simulink model "TSR_Scenario_002_cs"  (R2014b)
settings: Solver=ode5  SolverMode=SingleTasking  StartTime=0.0  StopTime=inf  FixedStep=1/100  RelTol=1e-3
PreLoadFcn:
  | mbxruntime.callbacks.PreLoadFcn(bdroot);
  | check_NUTS_defined;
  | 
  | assignin('base',['model_closed_' bdroot],false);
  | 
  | addpath('../includes_TSR/includes_TSR');
  | 
  | switch version('-release')
  | case {'2010a', '2010b', '2011a'}
  | addpath('../includes_TSR/ML2010b');
  | otherwise
  | addpath('../includes_TSR/ML2011b');
  | end
PostLoadFcn:
  | mbxruntime.callbacks.PostLoadFcn(bdroot);
InitFcn:
  | mbxruntime.callbacks.InitFcn(bdroot);;
  | 
  | addpath('..\includes_TSR');
StartFcn:
  | mbxruntime.callbacks.StartFcn(bdroot);
StopFcn:
  | mbxruntime.callbacks.StopFcn(bdroot);
model workspace: external: MAT-File .\TSR_Scenario_002_cs_hws.mat (data not in the file)
undefined symbols (not defined in the file or in its folder): InitImageOutputDir, mbxruntime, OrientationPitch, OrientationRoll, PositionX, PositionY, PositionZ, tabledata, warningInitialVelocity, x0
undefined symbols (not defined in the file): SteeringColumn, SteeringWheel, TSR_Scenario_002_cs_003e47b1b59594b6, TSR_Scenario_002_cs_023e87a31011dc74, TSR_Scenario_002_cs_048cb8409c90d9c6, TSR_Scenario_002_cs_106a0284aafa53e6, TSR_Scenario_002_cs_195b368d22a7f172, TSR_Scenario_002_cs_1e339fa5d680f213, TSR_Scenario_002_cs_26196a9fb104f950, TSR_Scenario_002_cs_261a709f6f453598, TSR_Scenario_002_cs_2ac3337370d0049d, TSR_Scenario_002_cs_2dc51e6a68b01b00, TSR_Scenario_002_cs_3460ff54d38ab2e2, TSR_Scenario_002_cs_42ea7d6e56bd6005, TSR_Scenario_002_cs_4dd419d6d2b56fc2, TSR_Scenario_002_cs_5316a21de09dff2f, TSR_Scenario_002_cs_538caacf3455966d, TSR_Scenario_002_cs_5b2cfdbcfc80811f, TSR_Scenario_002_cs_5ce0eafbb7a2dce7, TSR_Scenario_002_cs_62cdbf45c6f8824a, TSR_Scenario_002_cs_6bebc368eedff0bc, TSR_Scenario_002_cs_6d26481da4ed7e29, TSR_Scenario_002_cs_70c7e369ce6550e0, TSR_Scenario_002_cs_7a63051a1f311451, TSR_Scenario_002_cs_7d7dc8405f613c6d, TSR_Scenario_002_cs_7f65e296173485e8, TSR_Scenario_002_cs_87183cf6ff7bb4b6, TSR_Scenario_002_cs_8921b0da7ab80865, TSR_Scenario_002_cs_9495ce3a76763d1f, TSR_Scenario_002_cs_a679806a2fdc8099, TSR_Scenario_002_cs_Actros_1860_1_Path_pathUniqueID, TSR_Scenario_002_cs_Actros_2541_1_Path_pathUniqueID, TSR_Scenario_002_cs_Actros_2541_3_Path_pathUniqueID, TSR_Scenario_002_cs_Actros_2541_4_Path_pathUniqueID, TSR_Scenario_002_cs_adf24c93a9de8a4e, TSR_Scenario_002_cs_Audi_A8_1_Dynamics_Simple_initialPitch, TSR_Scenario_002_cs_Audi_A8_1_Dynamics_Simple_initialRoll, TSR_Scenario_002_cs_Audi_A8_1_Dynamics_Simple_initialX, TSR_Scenario_002_cs_Audi_A8_1_Dynamics_Simple_initialY, TSR_Scenario_002_cs_Audi_A8_1_Dynamics_Simple_initialYaw, TSR_Scenario_002_cs_Audi_A8_1_Dynamics_Simple_initialZ, TSR_Scenario_002_cs_b136c6ccb55f77db, TSR_Scenario_002_cs_ba4f809714c282b7, TSR_Scenario_002_cs_BMW_X5_1_Path_pathUniqueID, TSR_Scenario_002_cs_BMW_X5_1_SpeedProfile_speedProfileUniqueID, TSR_Scenario_002_cs_BMW_X5_2_Path_pathUniqueID, TSR_Scenario_002_cs_BMW_X5_2_SpeedProfile_speedProfileUniqueID, TSR_Scenario_002_cs_Citroen_C3_1_Path_pathUniqueID, TSR_Scenario_002_cs_Citroen_C3_2_Path_pathUniqueID, TSR_Scenario_002_cs_d8f275339b7082cf, TSR_Scenario_002_cs_Daf_95_1_Path_pathUniqueID, TSR_Scenario_002_cs_Daf_95_1_SpeedProfile_speedProfileUniqueID, TSR_Scenario_002_cs_dc019741510ce2f2, TSR_Scenario_002_cs_fdbc8aabe460b27c, TSR_Scenario_002_cs_Fiat_Bravo_1_Path_pathUniqueID, TSR_Scenario_002_cs_Ford_Fiesta_1_Path_pathUniqueID, TSR_Scenario_002_cs_Honda_Pan_European_1_Path_pathUniqueID, TSR_Scenario_002_cs_Mazda_RX8_1_Path_pathUniqueID, TSR_Scenario_002_cs_Nissan_Cabstar_1_Path_pathUniqueID, TSR_Scenario_002_cs_Nissan_Cabstar_2_Path_pathUniqueID ... (+9)
libraries: simulink_extras x82, simulink x23, PreScanSimulinkLibrary x11
(part 31 of 39)

== system TSR_Scenario_002_cs/VISUMatrixSign_HighwayOverhang_23/Actuator ==
  VISUMatrixSign_HighwayOverhang_23 : Inport  Tag=inport/VisuMatrixSign  SampleTime=1/100  BusOutputAsStruct=on
  DemuxVisuMatrixSign : Demux  Outputs=2
  visu_MatrixSign_13 : S-Function  FunctionName=sfun_ResourceNameSelector  Parameters=mbxruntime.parameters.convert(UniqueID), mbxruntime.parameters.convert(ResourceList), mbxruntime.parameters.convert(PivotName),tabledata, TimeStep  EnableBusSupport=off  mask(PreScan Sink Block: VisuMatrixSign){UniqueID=1102, ResourceList={'1' 'InformationSign\MatrixSign_GreenArrow.png' '2' 'InformationSign\Empty.jpeg' '3' 'InformationSign\SEARCH_Logo.png' '4' 'InformationSign\z274-50_black_full.png' '5' 'InformationSign\z274-51_black_full.png' '6' 'InformationSign\z274-52_black_full.png' '7' 'InformationSign\z274-53_black_full.png' '8' 'InformationSign\z274-54_black_full.png' '9' 'InformationSign\z274-55_black_full.png' '10' 'InformationSign\z274-56_black_full.png' '11' 'InformationSign\z274-57_black_full.png' '12' 'InformationSign\z274-58_black_full.png' '13' 'InformationSign\z274-59_black_full.png' '14' 'InformationSign\z274-60_black_full.png' '15' 'InformationSign\z274-61_black_full.png' '16' 'InformationSign\z274-62_black_full.png' '17' 'InformationSign\z274-63_black_full.png' }, PivotName=/child:name=MatrixSign_13/trafficSignElement, TimeStep=1/100}
      mask prompts: UniqueID "Parent Unique Identifier (auto-generated)"; ResourceList "Resource List (auto-generated)"; PivotName "Name of pivot (auto-generated)"; TimeStep "Simulink time step"
      mask help:
      | The VisuMatrixSign block provides a way to adapt the texture of the plates connected to an overhang, based on Resource IDs of the texture files.
      |
      | For more information, please click Help.
      mask init:
      | [tabledata] = mbxruntime.parameters.table(UniqueID,ResourceList,PivotName);
      mask Help: eval('openHelp(733)')
      mask Display: image(imread('HighwaySpeedMatrix.png'))
  visu_MatrixSign_54 : S-Function  FunctionName=sfun_ResourceNameSelector  Parameters=mbxruntime.parameters.convert(UniqueID), mbxruntime.parameters.convert(ResourceList), mbxruntime.parameters.convert(PivotName),tabledata, TimeStep  EnableBusSupport=off  mask(PreScan Sink Block: VisuMatrixSign){UniqueID=1102, ResourceList={'1' 'InformationSign\MatrixSign_GreenArrow.png' '2' 'InformationSign\Empty.jpeg' '3' 'InformationSign\SEARCH_Logo.png' '4' 'InformationSign\z274-50_black_full.png' '5' 'InformationSign\z274-51_black_full.png' '6' 'InformationSign\z274-52_black_full.png' '7' 'InformationSign\z274-53_black_full.png' '8' 'InformationSign\z274-54_black_full.png' '9' 'InformationSign\z274-55_black_full.png' '10' 'InformationSign\z274-56_black_full.png' '11' 'InformationSign\z274-57_black_full.png' '12' 'InformationSign\z274-58_black_full.png' '13' 'InformationSign\z274-59_black_full.png' '14' 'InformationSign\z274-60_black_full.png' '15' 'InformationSign\z274-61_black_full.png' '16' 'InformationSign\z274-62_black_full.png' '17' 'InformationSign\z274-63_black_full.png' }, PivotName=/child:name=MatrixSign_54/trafficSignElement, TimeStep=1/100}
      mask prompts: UniqueID "Parent Unique Identifier (auto-generated)"; ResourceList "Resource List (auto-generated)"; PivotName "Name of pivot (auto-generated)"; TimeStep "Simulink time step"
      mask help:
      | The VisuMatrixSign block provides a way to adapt the texture of the plates connected to an overhang, based on Resource IDs of the texture files.
      |
      | For more information, please click Help.
      mask init:
      | [tabledata] = mbxruntime.parameters.table(UniqueID,ResourceList,PivotName);
      mask Help: eval('openHelp(733)')
      mask Display: image(imread('HighwaySpeedMatrix.png'))
  wires:
  VISUMatrixSign_HighwayOverhang_23/1 -> DemuxVisuMatrixSign/1
  DemuxVisuMatrixSign/1 -> visu_MatrixSign_13/1
  DemuxVisuMatrixSign/2 -> visu_MatrixSign_54/1

== system TSR_Scenario_002_cs/VISUMatrixSign_HighwayOverhang_24/Actuator ==
  VISUMatrixSign_HighwayOverhang_24 : Inport  Tag=inport/VisuMatrixSign  SampleTime=1/100  BusOutputAsStruct=on
  DemuxVisuMatrixSign : Demux  Outputs=2
  visu_MatrixSign_25 : S-Function  FunctionName=sfun_ResourceNameSelector  Parameters=mbxruntime.parameters.convert(UniqueID), mbxruntime.parameters.convert(ResourceList), mbxruntime.parameters.convert(PivotName),tabledata, TimeStep  EnableBusSupport=off  mask(PreScan Sink Block: VisuMatrixSign){UniqueID=1103, ResourceList={'1' 'InformationSign\MatrixSign_GreenArrow.png' '2' 'InformationSign\Empty.jpeg' '3' 'InformationSign\SEARCH_Logo.png' '4' 'InformationSign\z274-50_black_full.png' '5' 'InformationSign\z274-51_black_full.png' '6' 'InformationSign\z274-52_black_full.png' '7' 'InformationSign\z274-53_black_full.png' '8' 'InformationSign\z274-54_black_full.png' '9' 'InformationSign\z274-55_black_full.png' '10' 'InformationSign\z274-56_black_full.png' '11' 'InformationSign\z274-57_black_full.png' '12' 'InformationSign\z274-58_black_full.png' '13' 'InformationSign\z274-59_black_full.png' '14' 'InformationSign\z274-60_black_full.png' '15' 'InformationSign\z274-61_black_full.png' '16' 'InformationSign\z274-62_black_full.png' '17' 'InformationSign\z274-63_black_full.png' }, PivotName=/child:name=MatrixSign_25/trafficSignElement, TimeStep=1/100}
      mask prompts: UniqueID "Parent Unique Identifier (auto-generated)"; ResourceList "Resource List (auto-generated)"; PivotName "Name of pivot (auto-generated)"; TimeStep "Simulink time step"
      mask help:
      | The VisuMatrixSign block provides a way to adapt the texture of the plates connected to an overhang, based on Resource IDs of the texture files.
      |
      | For more information, please click Help.
      mask init:
      | [tabledata] = mbxruntime.parameters.table(UniqueID,ResourceList,PivotName);
      mask Help: eval('openHelp(733)')
      mask Display: image(imread('HighwaySpeedMatrix.png'))
  visu_MatrixSign_55 : S-Function  FunctionName=sfun_ResourceNameSelector  Parameters=mbxruntime.parameters.convert(UniqueID), mbxruntime.parameters.convert(ResourceList), mbxruntime.parameters.convert(PivotName),tabledata, TimeStep  EnableBusSupport=off  mask(PreScan Sink Block: VisuMatrixSign){UniqueID=1103, ResourceList={'1' 'InformationSign\MatrixSign_GreenArrow.png' '2' 'InformationSign\Empty.jpeg' '3' 'InformationSign\SEARCH_Logo.png' '4' 'InformationSign\z274-50_black_full.png' '5' 'InformationSign\z274-51_black_full.png' '6' 'InformationSign\z274-52_black_full.png' '7' 'InformationSign\z274-53_black_full.png' '8' 'InformationSign\z274-54_black_full.png' '9' 'InformationSign\z274-55_black_full.png' '10' 'InformationSign\z274-56_black_full.png' '11' 'InformationSign\z274-57_black_full.png' '12' 'InformationSign\z274-58_black_full.png' '13' 'InformationSign\z274-59_black_full.png' '14' 'InformationSign\z274-60_black_full.png' '15' 'InformationSign\z274-61_black_full.png' '16' 'InformationSign\z274-62_black_full.png' '17' 'InformationSign\z274-63_black_full.png' }, PivotName=/child:name=MatrixSign_55/trafficSignElement, TimeStep=1/100}
      mask prompts: UniqueID "Parent Unique Identifier (auto-generated)"; ResourceList "Resource List (auto-generated)"; PivotName "Name of pivot (auto-generated)"; TimeStep "Simulink time step"
      mask help:
      | The VisuMatrixSign block provides a way to adapt the texture of the plates connected to an overhang, based on Resource IDs of the texture files.
      |
      | For more information, please click Help.
      mask init:
      | [tabledata] = mbxruntime.parameters.table(UniqueID,ResourceList,PivotName);
      mask Help: eval('openHelp(733)')
      mask Display: image(imread('HighwaySpeedMatrix.png'))
  wires:
  VISUMatrixSign_HighwayOverhang_24/1 -> DemuxVisuMatrixSign/1
  DemuxVisuMatrixSign/1 -> visu_MatrixSign_25/1
  DemuxVisuMatrixSign/2 -> visu_MatrixSign_55/1

== system TSR_Scenario_002_cs/VISUMatrixSign_HighwayOverhang_25/Actuator ==
  VISUMatrixSign_HighwayOverhang_25 : Inport  Tag=inport/VisuMatrixSign  SampleTime=1/100  BusOutputAsStruct=on
  DemuxVisuMatrixSign : Demux  Outputs=2
  visu_MatrixSign_26 : S-Function  FunctionName=sfun_ResourceNameSelector  Parameters=mbxruntime.parameters.convert(UniqueID), mbxruntime.parameters.convert(ResourceList), mbxruntime.parameters.convert(PivotName),tabledata, TimeStep  EnableBusSupport=off  mask(PreScan Sink Block: VisuMatrixSign){UniqueID=1104, ResourceList={'1' 'InformationSign\MatrixSign_GreenArrow.png' '2' 'InformationSign\Empty.jpeg' '3' 'InformationSign\SEARCH_Logo.png' '4' 'InformationSign\z274-50_black_full.png' '5' 'InformationSign\z274-51_black_full.png' '6' 'InformationSign\z274-52_black_full.png' '7' 'InformationSign\z274-53_black_full.png' '8' 'InformationSign\z274-54_black_full.png' '9' 'InformationSign\z274-55_black_full.png' '10' 'InformationSign\z274-56_black_full.png' '11' 'InformationSign\z274-57_black_full.png' '12' 'InformationSign\z274-58_black_full.png' '13' 'InformationSign\z274-59_black_full.png' '14' 'InformationSign\z274-60_black_full.png' '15' 'InformationSign\z274-61_black_full.png' '16' 'InformationSign\z274-62_black_full.png' '17' 'InformationSign\z274-63_black_full.png' }, PivotName=/child:name=MatrixSign_26/trafficSignElement, TimeStep=1/100}
      mask prompts: UniqueID "Parent Unique Identifier (auto-generated)"; ResourceList "Resource List (auto-generated)"; PivotName "Name of pivot (auto-generated)"; TimeStep "Simulink time step"
      mask help:
      | The VisuMatrixSign block provides a way to adapt the texture of the plates connected to an overhang, based on Resource IDs of the texture files.
      |
      | For more information, please click Help.
      mask init:
      | [tabledata] = mbxruntime.parameters.table(UniqueID,ResourceList,PivotName);
      mask Help: eval('openHelp(733)')
      mask Display: image(imread('HighwaySpeedMatrix.png'))
  visu_MatrixSign_56 : S-Function  FunctionName=sfun_ResourceNameSelector  Parameters=mbxruntime.parameters.convert(UniqueID), mbxruntime.parameters.convert(ResourceList), mbxruntime.parameters.convert(PivotName),tabledata, TimeStep  EnableBusSupport=off  mask(PreScan Sink Block: VisuMatrixSign){UniqueID=1104, ResourceList={'1' 'InformationSign\MatrixSign_GreenArrow.png' '2' 'InformationSign\Empty.jpeg' '3' 'InformationSign\SEARCH_Logo.png' '4' 'InformationSign\z274-50_black_full.png' '5' 'InformationSign\z274-51_black_full.png' '6' 'InformationSign\z274-52_black_full.png' '7' 'InformationSign\z274-53_black_full.png' '8' 'InformationSign\z274-54_black_full.png' '9' 'InformationSign\z274-55_black_full.png' '10' 'InformationSign\z274-56_black_full.png' '11' 'InformationSign\z274-57_black_full.png' '12' 'InformationSign\z274-58_black_full.png' '13' 'InformationSign\z274-59_black_full.png' '14' 'InformationSign\z274-60_black_full.png' '15' 'InformationSign\z274-61_black_full.png' '16' 'InformationSign\z274-62_black_full.png' '17' 'InformationSign\z274-63_black_full.png' }, PivotName=/child:name=MatrixSign_56/trafficSignElement, TimeStep=1/100}
      mask prompts: UniqueID "Parent Unique Identifier (auto-generated)"; ResourceList "Resource List (auto-generated)"; PivotName "Name of pivot (auto-generated)"; TimeStep "Simulink time step"
      mask help:
      | The VisuMatrixSign block provides a way to adapt the texture of the plates connected to an overhang, based on Resource IDs of the texture files.
      |
      | For more information, please click Help.
      mask init:
      | [tabledata] = mbxruntime.parameters.table(UniqueID,ResourceList,PivotName);
      mask Help: eval('openHelp(733)')
      mask Display: image(imread('HighwaySpeedMatrix.png'))
  wires:
  VISUMatrixSign_HighwayOverhang_25/1 -> DemuxVisuMatrixSign/1
  DemuxVisuMatrixSign/1 -> visu_MatrixSign_26/1
  DemuxVisuMatrixSign/2 -> visu_MatrixSign_56/1

== system TSR_Scenario_002_cs/VISUMatrixSign_HighwayOverhang_26/Actuator ==
  VISUMatrixSign_HighwayOverhang_26 : Inport  Tag=inport/VisuMatrixSign  SampleTime=1/100  BusOutputAsStruct=on
  DemuxVisuMatrixSign : Demux  Outputs=2
  visu_MatrixSign_37 : S-Function  FunctionName=sfun_ResourceNameSelector  Parameters=mbxruntime.parameters.convert(UniqueID), mbxruntime.parameters.convert(ResourceList), mbxruntime.parameters.convert(PivotName),tabledata, TimeStep  EnableBusSupport=off  mask(PreScan Sink Block: VisuMatrixSign){UniqueID=1105, ResourceList={'1' 'InformationSign\MatrixSign_GreenArrow.png' '2' 'InformationSign\Empty.jpeg' '3' 'InformationSign\SEARCH_Logo.png' '4' 'InformationSign\z274-50_black_full.png' '5' 'InformationSign\z274-51_black_full.png' '6' 'InformationSign\z274-52_black_full.png' '7' 'InformationSign\z274-53_black_full.png' '8' 'InformationSign\z274-54_black_full.png' '9' 'InformationSign\z274-55_black_full.png' '10' 'InformationSign\z274-56_black_full.png' '11' 'InformationSign\z274-57_black_full.png' '12' 'InformationSign\z274-58_black_full.png' '13' 'InformationSign\z274-59_black_full.png' '14' 'InformationSign\z274-60_black_full.png' '15' 'InformationSign\z274-61_black_full.png' '16' 'InformationSign\z274-62_black_full.png' '17' 'InformationSign\z274-63_black_full.png' }, PivotName=/child:name=MatrixSign_37/trafficSignElement, TimeStep=1/100}
      mask prompts: UniqueID "Parent Unique Identifier (auto-generated)"; ResourceList "Resource List (auto-generated)"; PivotName "Name of pivot (auto-generated)"; TimeStep "Simulink time step"
      mask help:
      | The VisuMatrixSign block provides a way to adapt the texture of the plates connected to an overhang, based on Resource IDs of the texture files.
      |
      | For more information, please click Help.
      mask init:
      | [tabledata] = mbxruntime.parameters.table(UniqueID,ResourceList,PivotName);
      mask Help: eval('openHelp(733)')
      mask Display: image(imread('HighwaySpeedMatrix.png'))
  visu_MatrixSign_38 : S-Function  FunctionName=sfun_ResourceNameSelector  Parameters=mbxruntime.parameters.convert(UniqueID), mbxruntime.parameters.convert(ResourceList), mbxruntime.parameters.convert(PivotName),tabledata, TimeStep  EnableBusSupport=off  mask(PreScan Sink Block: VisuMatrixSign){UniqueID=1105, ResourceList={'1' 'InformationSign\MatrixSign_GreenArrow.png' '2' 'InformationSign\Empty.jpeg' '3' 'InformationSign\SEARCH_Logo.png' '4' 'InformationSign\z274-50_black_full.png' '5' 'InformationSign\z274-51_black_full.png' '6' 'InformationSign\z274-52_black_full.png' '7' 'InformationSign\z274-53_black_full.png' '8' 'InformationSign\z274-54_black_full.png' '9' 'InformationSign\z274-55_black_full.png' '10' 'InformationSign\z274-56_black_full.png' '11' 'InformationSign\z274-57_black_full.png' '12' 'InformationSign\z274-58_black_full.png' '13' 'InformationSign\z274-59_black_full.png' '14' 'InformationSign\z274-60_black_full.png' '15' 'InformationSign\z274-61_black_full.png' '16' 'InformationSign\z274-62_black_full.png' '17' 'InformationSign\z274-63_black_full.png' }, PivotName=/child:name=MatrixSign_38/trafficSignElement, TimeStep=1/100}
      mask prompts: UniqueID "Parent Unique Identifier (auto-generated)"; ResourceList "Resource List (auto-generated)"; PivotName "Name of pivot (auto-generated)"; TimeStep "Simulink time step"
      mask help:
      | The VisuMatrixSign block provides a way to adapt the texture of the plates connected to an overhang, based on Resource IDs of the texture files.
      |
      | For more information, please click Help.
      mask init:
      | [tabledata] = mbxruntime.parameters.table(UniqueID,ResourceList,PivotName);
      mask Help: eval('openHelp(733)')
      mask Display: image(imread('HighwaySpeedMatrix.png'))
  wires:
  VISUMatrixSign_HighwayOverhang_26/1 -> DemuxVisuMatrixSign/1
  DemuxVisuMatrixSign/1 -> visu_MatrixSign_37/1
  DemuxVisuMatrixSign/2 -> visu_MatrixSign_38/1

== system TSR_Scenario_002_cs/VISUMatrixSign_HighwayOverhang_27/Actuator ==
  VISUMatrixSign_HighwayOverhang_27 : Inport  Tag=inport/VisuMatrixSign  SampleTime=1/100  BusOutputAsStruct=on
  DemuxVisuMatrixSign : Demux  Outputs=2
  visu_MatrixSign_39 : S-Function  FunctionName=sfun_ResourceNameSelector  Parameters=mbxruntime.parameters.convert(UniqueID), mbxruntime.parameters.convert(ResourceList), mbxruntime.parameters.convert(PivotName),tabledata, TimeStep  EnableBusSupport=off  mask(PreScan Sink Block: VisuMatrixSign){UniqueID=1106, ResourceList={'1' 'InformationSign\MatrixSign_GreenArrow.png' '2' 'InformationSign\Empty.jpeg' '3' 'InformationSign\SEARCH_Logo.png' '4' 'InformationSign\z274-50_black_full.png' '5' 'InformationSign\z274-51_black_full.png' '6' 'InformationSign\z274-52_black_full.png' '7' 'InformationSign\z274-53_black_full.png' '8' 'InformationSign\z274-54_black_full.png' '9' 'InformationSign\z274-55_black_full.png' '10' 'InformationSign\z274-56_black_full.png' '11' 'InformationSign\z274-57_black_full.png' '12' 'InformationSign\z274-58_black_full.png' '13' 'InformationSign\z274-59_black_full.png' '14' 'InformationSign\z274-60_black_full.png' '15' 'InformationSign\z274-61_black_full.png' '16' 'InformationSign\z274-62_black_full.png' '17' 'InformationSign\z274-63_black_full.png' }, PivotName=/child:name=MatrixSign_39/trafficSignElement, TimeStep=1/100}
      mask prompts: UniqueID "Parent Unique Identifier (auto-generated)"; ResourceList "Resource List (auto-generated)"; PivotName "Name of pivot (auto-generated)"; TimeStep "Simulink time step"
      mask help:
      | The VisuMatrixSign block provides a way to adapt the texture of the plates connected to an overhang, based on Resource IDs of the texture files.
      |
      | For more information, please click Help.
      mask init:
      | [tabledata] = mbxruntime.parameters.table(UniqueID,ResourceList,PivotName);
      mask Help: eval('openHelp(733)')
      mask Display: image(imread('HighwaySpeedMatrix.png'))
  visu_MatrixSign_40 : S-Function  FunctionName=sfun_ResourceNameSelector  Parameters=mbxruntime.parameters.convert(UniqueID), mbxruntime.parameters.convert(ResourceList), mbxruntime.parameters.convert(PivotName),tabledata, TimeStep  EnableBusSupport=off  mask(PreScan Sink Block: VisuMatrixSign){UniqueID=1106, ResourceList={'1' 'InformationSign\MatrixSign_GreenArrow.png' '2' 'InformationSign\Empty.jpeg' '3' 'InformationSign\SEARCH_Logo.png' '4' 'InformationSign\z274-50_black_full.png' '5' 'InformationSign\z274-51_black_full.png' '6' 'InformationSign\z274-52_black_full.png' '7' 'InformationSign\z274-53_black_full.png' '8' 'InformationSign\z274-54_black_full.png' '9' 'InformationSign\z274-55_black_full.png' '10' 'InformationSign\z274-56_black_full.png' '11' 'InformationSign\z274-57_black_full.png' '12' 'InformationSign\z274-58_black_full.png' '13' 'InformationSign\z274-59_black_full.png' '14' 'InformationSign\z274-60_black_full.png' '15' 'InformationSign\z274-61_black_full.png' '16' 'InformationSign\z274-62_black_full.png' '17' 'InformationSign\z274-63_black_full.png' }, PivotName=/child:name=MatrixSign_40/trafficSignElement, TimeStep=1/100}
      mask prompts: UniqueID "Parent Unique Identifier (auto-generated)"; ResourceList "Resource List (auto-generated)"; PivotName "Name of pivot (auto-generated)"; TimeStep "Simulink time step"
      mask help:
      | The VisuMatrixSign block provides a way to adapt the texture of the plates connected to an overhang, based on Resource IDs of the texture files.
      |
      | For more information, please click Help.
      mask init:
      | [tabledata] = mbxruntime.parameters.table(UniqueID,ResourceList,PivotName);
      mask Help: eval('openHelp(733)')
      mask Display: image(imread('HighwaySpeedMatrix.png'))
  wires:
  VISUMatrixSign_HighwayOverhang_27/1 -> DemuxVisuMatrixSign/1
  DemuxVisuMatrixSign/1 -> visu_MatrixSign_39/1
  DemuxVisuMatrixSign/2 -> visu_MatrixSign_40/1

== system TSR_Scenario_002_cs/VISUMatrixSign_HighwayOverhang_28/Actuator ==
  VISUMatrixSign_HighwayOverhang_28 : Inport  Tag=inport/VisuMatrixSign  SampleTime=1/100  BusOutputAsStruct=on
  DemuxVisuMatrixSign : Demux  Outputs=2
  visu_MatrixSign_41 : S-Function  FunctionName=sfun_ResourceNameSelector  Parameters=mbxruntime.parameters.convert(UniqueID), mbxruntime.parameters.convert(ResourceList), mbxruntime.parameters.convert(PivotName),tabledata, TimeStep  EnableBusSupport=off  mask(PreScan Sink Block: VisuMatrixSign){UniqueID=1107, ResourceList={'1' 'InformationSign\MatrixSign_GreenArrow.png' '2' 'InformationSign\Empty.jpeg' '3' 'InformationSign\SEARCH_Logo.png' '4' 'InformationSign\z274-50_black_full.png' '5' 'InformationSign\z274-51_black_full.png' '6' 'InformationSign\z274-52_black_full.png' '7' 'InformationSign\z274-53_black_full.png' '8' 'InformationSign\z274-54_black_full.png' '9' 'InformationSign\z274-55_black_full.png' '10' 'InformationSign\z274-56_black_full.png' '11' 'InformationSign\z274-57_black_full.png' '12' 'InformationSign\z274-58_black_full.png' '13' 'InformationSign\z274-59_black_full.png' '14' 'InformationSign\z274-60_black_full.png' '15' 'InformationSign\z274-61_black_full.png' '16' 'InformationSign\z274-62_black_full.png' '17' 'InformationSign\z274-63_black_full.png' }, PivotName=/child:name=MatrixSign_41/trafficSignElement, TimeStep=1/100}
      mask prompts: UniqueID "Parent Unique Identifier (auto-generated)"; ResourceList "Resource List (auto-generated)"; PivotName "Name of pivot (auto-generated)"; TimeStep "Simulink time step"
      mask help:
      | The VisuMatrixSign block provides a way to adapt the texture of the plates connected to an overhang, based on Resource IDs of the texture files.
      |
      | For more information, please click Help.
      mask init:
      | [tabledata] = mbxruntime.parameters.table(UniqueID,ResourceList,PivotName);
      mask Help: eval('openHelp(733)')
      mask Display: image(imread('HighwaySpeedMatrix.png'))
  visu_MatrixSign_42 : S-Function  FunctionName=sfun_ResourceNameSelector  Parameters=mbxruntime.parameters.convert(UniqueID), mbxruntime.parameters.convert(ResourceList), mbxruntime.parameters.convert(PivotName),tabledata, TimeStep  EnableBusSupport=off  mask(PreScan Sink Block: VisuMatrixSign){UniqueID=1107, ResourceList={'1' 'InformationSign\MatrixSign_GreenArrow.png' '2' 'InformationSign\Empty.jpeg' '3' 'InformationSign\SEARCH_Logo.png' '4' 'InformationSign\z274-50_black_full.png' '5' 'InformationSign\z274-51_black_full.png' '6' 'InformationSign\z274-52_black_full.png' '7' 'InformationSign\z274-53_black_full.png' '8' 'InformationSign\z274-54_black_full.png' '9' 'InformationSign\z274-55_black_full.png' '10' 'InformationSign\z274-56_black_full.png' '11' 'InformationSign\z274-57_black_full.png' '12' 'InformationSign\z274-58_black_full.png' '13' 'InformationSign\z274-59_black_full.png' '14' 'InformationSign\z274-60_black_full.png' '15' 'InformationSign\z274-61_black_full.png' '16' 'InformationSign\z274-62_black_full.png' '17' 'InformationSign\z274-63_black_full.png' }, PivotName=/child:name=MatrixSign_42/trafficSignElement, TimeStep=1/100}
      mask prompts: UniqueID "Parent Unique Identifier (auto-generated)"; ResourceList "Resource List (auto-generated)"; PivotName "Name of pivot (auto-generated)"; TimeStep "Simulink time step"
      mask help:
      | The VisuMatrixSign block provides a way to adapt the texture of the plates connected to an overhang, based on Resource IDs of the texture files.
      |
      | For more information, please click Help.
      mask init:
      | [tabledata] = mbxruntime.parameters.table(UniqueID,ResourceList,PivotName);
      mask Help: eval('openHelp(733)')
      mask Display: image(imread('HighwaySpeedMatrix.png'))
  wires:
  VISUMatrixSign_HighwayOverhang_28/1 -> DemuxVisuMatrixSign/1
  DemuxVisuMatrixSign/1 -> visu_MatrixSign_41/1
  DemuxVisuMatrixSign/2 -> visu_MatrixSign_42/1

== system TSR_Scenario_002_cs/VISUMatrixSign_HighwayOverhang_3/Actuator ==
  VISUMatrixSign_HighwayOverhang_3 : Inport  Tag=inport/VisuMatrixSign  SampleTime=1/100  BusOutputAsStruct=on
  DemuxVisuMatrixSign : Demux  Outputs=2
  visu_MatrixSign_12 : S-Function  FunctionName=sfun_ResourceNameSelector  Parameters=mbxruntime.parameters.convert(UniqueID), mbxruntime.parameters.convert(ResourceList), mbxruntime.parameters.convert(PivotName),tabledata, TimeStep  EnableBusSupport=off  mask(PreScan Sink Block: VisuMatrixSign){UniqueID=440, ResourceList={'1' 'InformationSign\MatrixSign_GreenArrow.png' '2' 'InformationSign\Empty.jpeg' '3' 'InformationSign\SEARCH_Logo.png' '4' 'InformationSign\z274-50_black_full.png' '5' 'InformationSign\z274-51_black_full.png' '6' 'InformationSign\z274-52_black_full.png' '7' 'InformationSign\z274-53_black_full.png' '8' 'InformationSign\z274-54_black_full.png' '9' 'InformationSign\z274-55_black_full.png' '10' 'InformationSign\z274-56_black_full.png' '11' 'InformationSign\z274-57_black_full.png' '12' 'InformationSign\z274-58_black_full.png' '13' 'InformationSign\z274-59_black_full.png' '14' 'InformationSign\z274-60_black_full.png' '15' 'InformationSign\z274-61_black_full.png' '16' 'InformationSign\z274-62_black_full.png' '17' 'InformationSign\z274-63_black_full.png' }, PivotName=/child:name=MatrixSign_12/trafficSignElement, TimeStep=1/100}
      mask prompts: UniqueID "Parent Unique Identifier (auto-generated)"; ResourceList "Resource List (auto-generated)"; PivotName "Name of pivot (auto-generated)"; TimeStep "Simulink time step"
      mask help:
      | The VisuMatrixSign block provides a way to adapt the texture of the plates connected to an overhang, based on Resource IDs of the texture files.
      |
      | For more information, please click Help.
      mask init:
      | [tabledata] = mbxruntime.parameters.table(UniqueID,ResourceList,PivotName);
      mask Help: eval('openHelp(733)')
      mask Display: image(imread('HighwaySpeedMatrix.png'))
  visu_MatrixSign_50 : S-Function  FunctionName=sfun_ResourceNameSelector  Parameters=mbxruntime.parameters.convert(UniqueID), mbxruntime.parameters.convert(ResourceList), mbxruntime.parameters.convert(PivotName),tabledata, TimeStep  EnableBusSupport=off  mask(PreScan Sink Block: VisuMatrixSign){UniqueID=440, ResourceList={'1' 'InformationSign\MatrixSign_GreenArrow.png' '2' 'InformationSign\Empty.jpeg' '3' 'InformationSign\SEARCH_Logo.png' '4' 'InformationSign\z274-50_black_full.png' '5' 'InformationSign\z274-51_black_full.png' '6' 'InformationSign\z274-52_black_full.png' '7' 'InformationSign\z274-53_black_full.png' '8' 'InformationSign\z274-54_black_full.png' '9' 'InformationSign\z274-55_black_full.png' '10' 'InformationSign\z274-56_black_full.png' '11' 'InformationSign\z274-57_black_full.png' '12' 'InformationSign\z274-58_black_full.png' '13' 'InformationSign\z274-59_black_full.png' '14' 'InformationSign\z274-60_black_full.png' '15' 'InformationSign\z274-61_black_full.png' '16' 'InformationSign\z274-62_black_full.png' '17' 'InformationSign\z274-63_black_full.png' }, PivotName=/child:name=MatrixSign_50/trafficSignElement, TimeStep=1/100}
      mask prompts: UniqueID "Parent Unique Identifier (auto-generated)"; ResourceList "Resource List (auto-generated)"; PivotName "Name of pivot (auto-generated)"; TimeStep "Simulink time step"
      mask help:
      | The VisuMatrixSign block provides a way to adapt the texture of the plates connected to an overhang, based on Resource IDs of the texture files.
      |
      | For more information, please click Help.
      mask init:
      | [tabledata] = mbxruntime.parameters.table(UniqueID,ResourceList,PivotName);
      mask Help: eval('openHelp(733)')
      mask Display: image(imread('HighwaySpeedMatrix.png'))
  wires:
  VISUMatrixSign_HighwayOverhang_3/1 -> DemuxVisuMatrixSign/1
  DemuxVisuMatrixSign/1 -> visu_MatrixSign_12/1
  DemuxVisuMatrixSign/2 -> visu_MatrixSign_50/1

== system TSR_Scenario_002_cs/VISUMatrixSign_HighwayOverhang_4/Actuator ==
  VISUMatrixSign_HighwayOverhang_4 : Inport  Tag=inport/VisuMatrixSign  SampleTime=1/100  BusOutputAsStruct=on
  DemuxVisuMatrixSign : Demux  Outputs=2
  visu_MatrixSign_23 : S-Function  FunctionName=sfun_ResourceNameSelector  Parameters=mbxruntime.parameters.convert(UniqueID), mbxruntime.parameters.convert(ResourceList), mbxruntime.parameters.convert(PivotName),tabledata, TimeStep  EnableBusSupport=off  mask(PreScan Sink Block: VisuMatrixSign){UniqueID=441, ResourceList={'1' 'InformationSign\MatrixSign_GreenArrow.png' '2' 'InformationSign\Empty.jpeg' '3' 'InformationSign\SEARCH_Logo.png' '4' 'InformationSign\z274-50_black_full.png' '5' 'InformationSign\z274-51_black_full.png' '6' 'InformationSign\z274-52_black_full.png' '7' 'InformationSign\z274-53_black_full.png' '8' 'InformationSign\z274-54_black_full.png' '9' 'InformationSign\z274-55_black_full.png' '10' 'InformationSign\z274-56_black_full.png' '11' 'InformationSign\z274-57_black_full.png' '12' 'InformationSign\z274-58_black_full.png' '13' 'InformationSign\z274-59_black_full.png' '14' 'InformationSign\z274-60_black_full.png' '15' 'InformationSign\z274-61_black_full.png' '16' 'InformationSign\z274-62_black_full.png' '17' 'InformationSign\z274-63_black_full.png' }, PivotName=/child:name=MatrixSign_23/trafficSignElement, TimeStep=1/100}
      mask prompts: UniqueID "Parent Unique Identifier (auto-generated)"; ResourceList "Resource List (auto-generated)"; PivotName "Name of pivot (auto-generated)"; TimeStep "Simulink time step"
      mask help:
      | The VisuMatrixSign block provides a way to adapt the texture of the plates connected to an overhang, based on Resource IDs of the texture files.
      |
      | For more information, please click Help.
      mask init:
      | [tabledata] = mbxruntime.parameters.table(UniqueID,ResourceList,PivotName);
      mask Help: eval('openHelp(733)')
      mask Display: image(imread('HighwaySpeedMatrix.png'))
  visu_MatrixSign_24 : S-Function  FunctionName=sfun_ResourceNameSelector  Parameters=mbxruntime.parameters.convert(UniqueID), mbxruntime.parameters.convert(ResourceList), mbxruntime.parameters.convert(PivotName),tabledata, TimeStep  EnableBusSupport=off  mask(PreScan Sink Block: VisuMatrixSign){UniqueID=441, ResourceList={'1' 'InformationSign\MatrixSign_GreenArrow.png' '2' 'InformationSign\Empty.jpeg' '3' 'InformationSign\SEARCH_Logo.png' '4' 'InformationSign\z274-50_black_full.png' '5' 'InformationSign\z274-51_black_full.png' '6' 'InformationSign\z274-52_black_full.png' '7' 'InformationSign\z274-53_black_full.png' '8' 'InformationSign\z274-54_black_full.png' '9' 'InformationSign\z274-55_black_full.png' '10' 'InformationSign\z274-56_black_full.png' '11' 'InformationSign\z274-57_black_full.png' '12' 'InformationSign\z274-58_black_full.png' '13' 'InformationSign\z274-59_black_full.png' '14' 'InformationSign\z274-60_black_full.png' '15' 'InformationSign\z274-61_black_full.png' '16' 'InformationSign\z274-62_black_full.png' '17' 'InformationSign\z274-63_black_full.png' }, PivotName=/child:name=MatrixSign_24/trafficSignElement, TimeStep=1/100}
      mask prompts: UniqueID "Parent Unique Identifier (auto-generated)"; ResourceList "Resource List (auto-generated)"; PivotName "Name of pivot (auto-generated)"; TimeStep "Simulink time step"
      mask help:
      | The VisuMatrixSign block provides a way to adapt the texture of the plates connected to an overhang, based on Resource IDs of the texture files.
      |
      | For more information, please click Help.
      mask init:
      | [tabledata] = mbxruntime.parameters.table(UniqueID,ResourceList,PivotName);
      mask Help: eval('openHelp(733)')
      mask Display: image(imread('HighwaySpeedMatrix.png'))
  wires:
  VISUMatrixSign_HighwayOverhang_4/1 -> DemuxVisuMatrixSign/1
  DemuxVisuMatrixSign/1 -> visu_MatrixSign_23/1
  DemuxVisuMatrixSign/2 -> visu_MatrixSign_24/1

== system TSR_Scenario_002_cs/VISUMatrixSign_HighwayOverhang_5/Actuator ==
  VISUMatrixSign_HighwayOverhang_5 : Inport  Tag=inport/VisuMatrixSign  SampleTime=1/100  BusOutputAsStruct=on
  DemuxVisuMatrixSign : Demux  Outputs=2
  visu_MatrixSign_48 : S-Function  FunctionName=sfun_ResourceNameSelector  Parameters=mbxruntime.parameters.convert(UniqueID), mbxruntime.parameters.convert(ResourceList), mbxruntime.parameters.convert(PivotName),tabledata, TimeStep  EnableBusSupport=off  mask(PreScan Sink Block: VisuMatrixSign){UniqueID=843, ResourceList={'1' 'InformationSign\MatrixSign_GreenArrow.png' '2' 'InformationSign\Empty.jpeg' '3' 'InformationSign\SEARCH_Logo.png' '4' 'InformationSign\z274-50_black_full.png' '5' 'InformationSign\z274-51_black_full.png' '6' 'InformationSign\z274-52_black_full.png' '7' 'InformationSign\z274-53_black_full.png' '8' 'InformationSign\z274-54_black_full.png' '9' 'InformationSign\z274-55_black_full.png' '10' 'InformationSign\z274-56_black_full.png' '11' 'InformationSign\z274-57_black_full.png' '12' 'InformationSign\z274-58_black_full.png' '13' 'InformationSign\z274-59_black_full.png' '14' 'InformationSign\z274-60_black_full.png' '15' 'InformationSign\z274-61_black_full.png' '16' 'InformationSign\z274-62_black_full.png' '17' 'InformationSign\z274-63_black_full.png' }, PivotName=/child:name=MatrixSign_48/trafficSignElement, TimeStep=1/100}
      mask prompts: UniqueID "Parent Unique Identifier (auto-generated)"; ResourceList "Resource List (auto-generated)"; PivotName "Name of pivot (auto-generated)"; TimeStep "Simulink time step"
      mask help:
      | The VisuMatrixSign block provides a way to adapt the texture of the plates connected to an overhang, based on Resource IDs of the texture files.
      |
      | For more information, please click Help.
      mask init:
      | [tabledata] = mbxruntime.parameters.table(UniqueID,ResourceList,PivotName);
      mask Help: eval('openHelp(733)')
      mask Display: image(imread('HighwaySpeedMatrix.png'))
  visu_MatrixSign_8 : S-Function  FunctionName=sfun_ResourceNameSelector  Parameters=mbxruntime.parameters.convert(UniqueID), mbxruntime.parameters.convert(ResourceList), mbxruntime.parameters.convert(PivotName),tabledata, TimeStep  EnableBusSupport=off  mask(PreScan Sink Block: VisuMatrixSign){UniqueID=843, ResourceList={'1' 'InformationSign\MatrixSign_GreenArrow.png' '2' 'InformationSign\Empty.jpeg' '3' 'InformationSign\SEARCH_Logo.png' '4' 'InformationSign\z274-50_black_full.png' '5' 'InformationSign\z274-51_black_full.png' '6' 'InformationSign\z274-52_black_full.png' '7' 'InformationSign\z274-53_black_full.png' '8' 'InformationSign\z274-54_black_full.png' '9' 'InformationSign\z274-55_black_full.png' '10' 'InformationSign\z274-56_black_full.png' '11' 'InformationSign\z274-57_black_full.png' '12' 'InformationSign\z274-58_black_full.png' '13' 'InformationSign\z274-59_black_full.png' '14' 'InformationSign\z274-60_black_full.png' '15' 'InformationSign\z274-61_black_full.png' '16' 'InformationSign\z274-62_black_full.png' '17' 'InformationSign\z274-63_black_full.png' }, PivotName=/child:name=MatrixSign_8/trafficSignElement, TimeStep=1/100}
      mask prompts: UniqueID "Parent Unique Identifier (auto-generated)"; ResourceList "Resource List (auto-generated)"; PivotName "Name of pivot (auto-generated)"; TimeStep "Simulink time step"
      mask help:
      | The VisuMatrixSign block provides a way to adapt the texture of the plates connected to an overhang, based on Resource IDs of the texture files.
      |
      | For more information, please click Help.
      mask init:
      | [tabledata] = mbxruntime.parameters.table(UniqueID,ResourceList,PivotName);
      mask Help: eval('openHelp(733)')
      mask Display: image(imread('HighwaySpeedMatrix.png'))
  wires:
  VISUMatrixSign_HighwayOverhang_5/1 -> DemuxVisuMatrixSign/1
  DemuxVisuMatrixSign/1 -> visu_MatrixSign_8/1
  DemuxVisuMatrixSign/2 -> visu_MatrixSign_48/1

== system TSR_Scenario_002_cs/VISUMatrixSign_HighwayOverhang_6/Actuator ==
  VISUMatrixSign_HighwayOverhang_6 : Inport  Tag=inport/VisuMatrixSign  SampleTime=1/100  BusOutputAsStruct=on
  DemuxVisuMatrixSign : Demux  Outputs=2
  visu_MatrixSign_19 : S-Function  FunctionName=sfun_ResourceNameSelector  Parameters=mbxruntime.parameters.convert(UniqueID), mbxruntime.parameters.convert(ResourceList), mbxruntime.parameters.convert(PivotName),tabledata, TimeStep  EnableBusSupport=off  mask(PreScan Sink Block: VisuMatrixSign){UniqueID=846, ResourceList={'1' 'InformationSign\MatrixSign_GreenArrow.png' '2' 'InformationSign\Empty.jpeg' '3' 'InformationSign\SEARCH_Logo.png' '4' 'InformationSign\z274-50_black_full.png' '5' 'InformationSign\z274-51_black_full.png' '6' 'InformationSign\z274-52_black_full.png' '7' 'InformationSign\z274-53_black_full.png' '8' 'InformationSign\z274-54_black_full.png' '9' 'InformationSign\z274-55_black_full.png' '10' 'InformationSign\z274-56_black_full.png' '11' 'InformationSign\z274-57_black_full.png' '12' 'InformationSign\z274-58_black_full.png' '13' 'InformationSign\z274-59_black_full.png' '14' 'InformationSign\z274-60_black_full.png' '15' 'InformationSign\z274-61_black_full.png' '16' 'InformationSign\z274-62_black_full.png' '17' 'InformationSign\z274-63_black_full.png' }, PivotName=/child:name=MatrixSign_19/trafficSignElement, TimeStep=1/100}
      mask prompts: UniqueID "Parent Unique Identifier (auto-generated)"; ResourceList "Resource List (auto-generated)"; PivotName "Name of pivot (auto-generated)"; TimeStep "Simulink time step"
      mask help:
      | The VisuMatrixSign block provides a way to adapt the texture of the plates connected to an overhang, based on Resource IDs of the texture files.
      |
      | For more information, please click Help.
      mask init:
      | [tabledata] = mbxruntime.parameters.table(UniqueID,ResourceList,PivotName);
      mask Help: eval('openHelp(733)')
      mask Display: image(imread('HighwaySpeedMatrix.png'))
  visu_MatrixSign_20 : S-Function  FunctionName=sfun_ResourceNameSelector  Parameters=mbxruntime.parameters.convert(UniqueID), mbxruntime.parameters.convert(ResourceList), mbxruntime.parameters.convert(PivotName),tabledata, TimeStep  EnableBusSupport=off  mask(PreScan Sink Block: VisuMatrixSign){UniqueID=846, ResourceList={'1' 'InformationSign\MatrixSign_GreenArrow.png' '2' 'InformationSign\Empty.jpeg' '3' 'InformationSign\SEARCH_Logo.png' '4' 'InformationSign\z274-50_black_full.png' '5' 'InformationSign\z274-51_black_full.png' '6' 'InformationSign\z274-52_black_full.png' '7' 'InformationSign\z274-53_black_full.png' '8' 'InformationSign\z274-54_black_full.png' '9' 'InformationSign\z274-55_black_full.png' '10' 'InformationSign\z274-56_black_full.png' '11' 'InformationSign\z274-57_black_full.png' '12' 'InformationSign\z274-58_black_full.png' '13' 'InformationSign\z274-59_black_full.png' '14' 'InformationSign\z274-60_black_full.png' '15' 'InformationSign\z274-61_black_full.png' '16' 'InformationSign\z274-62_black_full.png' '17' 'InformationSign\z274-63_black_full.png' }, PivotName=/child:name=MatrixSign_20/trafficSignElement, TimeStep=1/100}
      mask prompts: UniqueID "Parent Unique Identifier (auto-generated)"; ResourceList "Resource List (auto-generated)"; PivotName "Name of pivot (auto-generated)"; TimeStep "Simulink time step"
      mask help:
      | The VisuMatrixSign block provides a way to adapt the texture of the plates connected to an overhang, based on Resource IDs of the texture files.
      |
      | For more information, please click Help.
      mask init:
      | [tabledata] = mbxruntime.parameters.table(UniqueID,ResourceList,PivotName);
      mask Help: eval('openHelp(733)')
      mask Display: image(imread('HighwaySpeedMatrix.png'))
  wires:
  VISUMatrixSign_HighwayOverhang_6/1 -> DemuxVisuMatrixSign/1
  DemuxVisuMatrixSign/1 -> visu_MatrixSign_19/1
  DemuxVisuMatrixSign/2 -> visu_MatrixSign_20/1

== system TSR_Scenario_002_cs/VISUMatrixSign_HighwayOverhang_7/Actuator ==
  VISUMatrixSign_HighwayOverhang_7 : Inport  Tag=inport/VisuMatrixSign  SampleTime=1/100  BusOutputAsStruct=on
  DemuxVisuMatrixSign : Demux  Outputs=2
  visu_MatrixSign_4 : S-Function  FunctionName=sfun_ResourceNameSelector  Parameters=mbxruntime.parameters.convert(UniqueID), mbxruntime.parameters.convert(ResourceList), mbxruntime.parameters.convert(PivotName),tabledata, TimeStep  EnableBusSupport=off  mask(PreScan Sink Block: VisuMatrixSign){UniqueID=867, ResourceList={'1' 'InformationSign\MatrixSign_GreenArrow.png' '2' 'InformationSign\Empty.jpeg' '3' 'InformationSign\SEARCH_Logo.png' '4' 'InformationSign\z274-50_black_full.png' '5' 'InformationSign\z274-51_black_full.png' '6' 'InformationSign\z274-52_black_full.png' '7' 'InformationSign\z274-53_black_full.png' '8' 'InformationSign\z274-54_black_full.png' '9' 'InformationSign\z274-55_black_full.png' '10' 'InformationSign\z274-56_black_full.png' '11' 'InformationSign\z274-57_black_full.png' '12' 'InformationSign\z274-58_black_full.png' '13' 'InformationSign\z274-59_black_full.png' '14' 'InformationSign\z274-60_black_full.png' '15' 'InformationSign\z274-61_black_full.png' '16' 'InformationSign\z274-62_black_full.png' '17' 'InformationSign\z274-63_black_full.png' }, PivotName=/child:name=MatrixSign_4/trafficSignElement, TimeStep=1/100}
      mask prompts: UniqueID "Parent Unique Identifier (auto-generated)"; ResourceList "Resource List (auto-generated)"; PivotName "Name of pivot (auto-generated)"; TimeStep "Simulink time step"
      mask help:
      | The VisuMatrixSign block provides a way to adapt the texture of the plates connected to an overhang, based on Resource IDs of the texture files.
      |
      | For more information, please click Help.
      mask init:
      | [tabledata] = mbxruntime.parameters.table(UniqueID,ResourceList,PivotName);
      mask Help: eval('openHelp(733)')
      mask Display: image(imread('HighwaySpeedMatrix.png'))
  visu_MatrixSign_45 : S-Function  FunctionName=sfun_ResourceNameSelector  Parameters=mbxruntime.parameters.convert(UniqueID), mbxruntime.parameters.convert(ResourceList), mbxruntime.parameters.convert(PivotName),tabledata, TimeStep  EnableBusSupport=off  mask(PreScan Sink Block: VisuMatrixSign){UniqueID=867, ResourceList={'1' 'InformationSign\MatrixSign_GreenArrow.png' '2' 'InformationSign\Empty.jpeg' '3' 'InformationSign\SEARCH_Logo.png' '4' 'InformationSign\z274-50_black_full.png' '5' 'InformationSign\z274-51_black_full.png' '6' 'InformationSign\z274-52_black_full.png' '7' 'InformationSign\z274-53_black_full.png' '8' 'InformationSign\z274-54_black_full.png' '9' 'InformationSign\z274-55_black_full.png' '10' 'InformationSign\z274-56_black_full.png' '11' 'InformationSign\z274-57_black_full.png' '12' 'InformationSign\z274-58_black_full.png' '13' 'InformationSign\z274-59_black_full.png' '14' 'InformationSign\z274-60_black_full.png' '15' 'InformationSign\z274-61_black_full.png' '16' 'InformationSign\z274-62_black_full.png' '17' 'InformationSign\z274-63_black_full.png' }, PivotName=/child:name=MatrixSign_45/trafficSignElement, TimeStep=1/100}
      mask prompts: UniqueID "Parent Unique Identifier (auto-generated)"; ResourceList "Resource List (auto-generated)"; PivotName "Name of pivot (auto-generated)"; TimeStep "Simulink time step"
      mask help:
      | The VisuMatrixSign block provides a way to adapt the texture of the plates connected to an overhang, based on Resource IDs of the texture files.
      |
      | For more information, please click Help.
      mask init:
      | [tabledata] = mbxruntime.parameters.table(UniqueID,ResourceList,PivotName);
      mask Help: eval('openHelp(733)')
      mask Display: image(imread('HighwaySpeedMatrix.png'))
  wires:
  VISUMatrixSign_HighwayOverhang_7/1 -> DemuxVisuMatrixSign/1
  DemuxVisuMatrixSign/1 -> visu_MatrixSign_4/1
  DemuxVisuMatrixSign/2 -> visu_MatrixSign_45/1
